simulink model "Speed"  (R2021a)
settings: Solver=ode113  StartTime=0.0  StopTime=1  RelTol=1e-6
model workspace (MAT data in the model file):
  Vdc = 30
  f_pwm = 10000
libraries: pid_lib x7, spsControlledVoltageSourceLib x2, spsGroundLib x2, spsPermanentMagnetSynchronousMachineLib x2, spsThreePhaseVIMeasurementLib x2, spsUniversalBridgeLib x2, spsTriangleGeneratorLib x2, spspowerguiLib x1
settings Model: SimulationMode=accelerator  Creator=Zzx  LastModifiedBy=Zzx
settings SolverCC: ZeroCrossAlgorithm=Adaptive

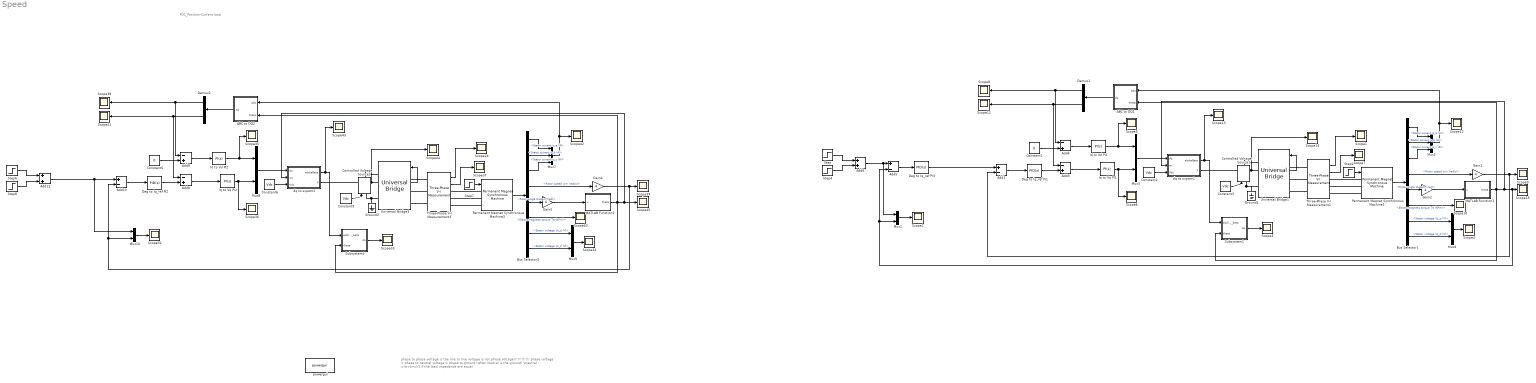
== system Speed ==
  note: FOC_Position-Current loop
  note: phase to phase voltage is the line to line voltage
      | is not phase voltage!!!!!!!!!!!!
      | phase voltage = phase to neutral voltage = phase to ground (when neutral is the ground)
      | Vneutral =(a+b+c)/3 if the load impedance are equal
  ABC to DQ1 : Subsystem
  ABC to DQ2 : Subsystem
  Add1 : Sum  Inputs=+-
  Add10 : Sum  Inputs=+-
  Add11 : Sum
  Add{3..4,8..9} (4 alike) : Sum  Inputs=-+
  Add5 : Sum  Inputs=+-
  Add6 : Sum
  Bus Selector1 : BusSelector  OutputSignals=Stator current is_a (A),Stator current is_b (A),Stator current is_c (A),Rotor speed wm (rad/s),Rotor angle thetam (rad),Electromagnetic torque Te (N*m),Stator voltage Vs_q (V),Stator voltage Vs_d (V)
  Bus Selector3 : BusSelector  OutputSignals=Stator current is_a (A),Stator current is_b (A),Stator current is_c (A),Rotor speed wm (rad/s),Rotor angle thetam (rad),Electromagnetic torque Te (N*m),Stator voltage Vs_q (V),Stator voltage Vs_d (V)
  Constant1 : Constant  Value=0
  Constant{2..3,6,9} (4 alike) : Constant  Value=Vdc
  Constant5 : Constant  Value=0
  Controlled Voltage Source1 : spsControlledVoltageSourceLib/Controlled Voltage Source  Initialize=on  Source_Type=DC  Amplitude=0  Phase=0  Frequency=0  Measurements=Voltage
  Controlled Voltage Source2 : spsControlledVoltageSourceLib/Controlled Voltage Source  Initialize=on  Source_Type=DC  Amplitude=0  Phase=0  Frequency=0  Measurements=Voltage
  Deg to Iq_ref PI1 : pid_lib/PID Controller  Controller=PID  Form=Parallel  TimeDomain=Continuous-time  UseExternalTs=off  SampleTime=-1  IntegratorMethod=Forward Euler  FilterMethod=Forward Euler  ControllerParametersSource=internal  P=80  I=0.1  D=1  UseFilter=on  N=10  TunerSelectOption=Frequency Response Based  InitialConditionSource=internal  InitialConditionForIntegrator=0  InitialConditionForFilter=0  DifferentiatorICPrevScaledInput=0  ExternalReset=none  TrackingMode=off  Kt=1  LimitOutput=off  SatLimitsSource=internal  UpperSaturationLimit=inf  LowerSaturationLimit=-inf  LinearizeAsGain=on  AntiWindupMode=none  Kb=1  POutMin=[]  POutMax=[]  IOutMin=[]  IOutMax=[]  DOutMin=[]  DOutMax=[]  NOutMin=[]  NOutMax=[]  SumOutMin=[]  SumOutMax=[]  SaturationOutMin=[]  SaturationOutMax=[]  PParamMin=[]  PParamMax=[]  IParamMin=[]  IParamMax=[]  DParamMin=[]  DParamMax=[]  NParamMin=[]  NParamMax=[]  KbParamMin=[]  KbParamMax=[]  KtParamMin=[]  KtParamMax=[]  KbOutMin=[]  KbOutMax=[]  KtOutMin=[]  KtOutMax=[]  IntegratorOutMin=[]  IntegratorOutMax=[]  FilterOutMin=[]  FilterOutMax=[]  SumI1OutMin=[]  SumI1OutMax=[]  SumI2OutMin=[]  SumI2OutMax=[]  SumI3OutMin=[]  SumI3OutMax=[]  SumI4OutMin=[]  SumI4OutMax=[]  SumDOutMin=[]  SumDOutMax=[]  DifferentiatorOutMin=[]  DifferentiatorOutMax=[]  FilterDiffOutCoefMin=[]  FilterDiffOutCoefMax=[]  ReciprocalOutMin=[]  ReciprocalOutMax=[]  SumDenOutMin=[]  SumDenOutMax=[]  SumNumOutMin=[]  SumNumOutMax=[]  DivideOutMin=[]  DivideOutMax=[]  UdiffTsProdOutMin=[]  UdiffTsProdOutMax=[]  NTsProdOutMin=[]  NTsProdOutMax=[]  UintegralTsProdOutMin=[]  UintegralTsProdOutMax=[]  UngainTsProdOutMin=[]  UngainTsProdOutMax=[]  IntegratorContinuousStateAttributes=''  IntegratorStateMustResolveToSignalObject=off  IntegratorRTWStateStorageClass=Auto  FilterContinuousStateAttributes=''  FilterStateMustResolveToSignalObject=off  FilterRTWStateStorageClass=Auto  ParallelPVariant=InternalParameters  IdealPVariant=Disabled  IVariant=InternalParameters  DVariant=InternalParameters  IntegratorVariant=Continuous  SatVariant=Disabled  AWVariant=Passthrough  PCopyVariant=Disabled  TRVariant=Disabled  FdbkBlocksVariant=Forward  IdealPFdbkVariant=Disabled  SatFdbkVariant=Disabled  DerivativeFilterVariant=ContFilter  NVariant=InternalParameters  NCopyVariant=Disabled  FilterICVariant=InternalICsFilter  IntegratorICVariant=InternalICs  ExternalResetVariant=Disabled  TRSumVariant=Passthrough  SumFdbkVariant=Disabled  SumVariant=Sum_PID  TsampFilterVariant=InternalTs  TsampNgainVariant=Passthrough  TsampIntegralVariant=Passthrough  ExternalSaturationOutDataTypeStr=Inherit: Same as second input
  Deg to Iq_ref PI2 : pid_lib/PID Controller  Controller=PID  Form=Parallel  TimeDomain=Continuous-time  UseExternalTs=off  SampleTime=-1  IntegratorMethod=Forward Euler  FilterMethod=Forward Euler  ControllerParametersSource=internal  P=80  I=0.1  D=0.1  UseFilter=on  N=10  TunerSelectOption=Frequency Response Based  InitialConditionSource=internal  InitialConditionForIntegrator=0  InitialConditionForFilter=0  DifferentiatorICPrevScaledInput=0  ExternalReset=none  TrackingMode=off  Kt=1  LimitOutput=off  SatLimitsSource=internal  UpperSaturationLimit=inf  LowerSaturationLimit=-inf  LinearizeAsGain=on  AntiWindupMode=none  Kb=1  POutMin=[]  POutMax=[]  IOutMin=[]  IOutMax=[]  DOutMin=[]  DOutMax=[]  NOutMin=[]  NOutMax=[]  SumOutMin=[]  SumOutMax=[]  SaturationOutMin=[]  SaturationOutMax=[]  PParamMin=[]  PParamMax=[]  IParamMin=[]  IParamMax=[]  DParamMin=[]  DParamMax=[]  NParamMin=[]  NParamMax=[]  KbParamMin=[]  KbParamMax=[]  KtParamMin=[]  KtParamMax=[]  KbOutMin=[]  KbOutMax=[]  KtOutMin=[]  KtOutMax=[]  IntegratorOutMin=[]  IntegratorOutMax=[]  FilterOutMin=[]  FilterOutMax=[]  SumI1OutMin=[]  SumI1OutMax=[]  SumI2OutMin=[]  SumI2OutMax=[]  SumI3OutMin=[]  SumI3OutMax=[]  SumI4OutMin=[]  SumI4OutMax=[]  SumDOutMin=[]  SumDOutMax=[]  DifferentiatorOutMin=[]  DifferentiatorOutMax=[]  FilterDiffOutCoefMin=[]  FilterDiffOutCoefMax=[]  ReciprocalOutMin=[]  ReciprocalOutMax=[]  SumDenOutMin=[]  SumDenOutMax=[]  SumNumOutMin=[]  SumNumOutMax=[]  DivideOutMin=[]  DivideOutMax=[]  UdiffTsProdOutMin=[]  UdiffTsProdOutMax=[]  NTsProdOutMin=[]  NTsProdOutMax=[]  UintegralTsProdOutMin=[]  UintegralTsProdOutMax=[]  UngainTsProdOutMin=[]  UngainTsProdOutMax=[]  IntegratorContinuousStateAttributes=''  IntegratorStateMustResolveToSignalObject=off  IntegratorRTWStateStorageClass=Auto  FilterContinuousStateAttributes=''  FilterStateMustResolveToSignalObject=off  FilterRTWStateStorageClass=Auto  ParallelPVariant=InternalParameters  IdealPVariant=Disabled  IVariant=InternalParameters  DVariant=InternalParameters  IntegratorVariant=Continuous  SatVariant=Disabled  AWVariant=Passthrough  PCopyVariant=Disabled  TRVariant=Disabled  FdbkBlocksVariant=Forward  IdealPFdbkVariant=Disabled  SatFdbkVariant=Disabled  DerivativeFilterVariant=ContFilter  NVariant=InternalParameters  NCopyVariant=Disabled  FilterICVariant=InternalICsFilter  IntegratorICVariant=InternalICs  ExternalResetVariant=Disabled  TRSumVariant=Passthrough  SumFdbkVariant=Disabled  SumVariant=Sum_PID  TsampFilterVariant=InternalTs  TsampNgainVariant=Passthrough  TsampIntegralVariant=Passthrough  ExternalSaturationOutDataTypeStr=Inherit: Same as second input
  Deg to Iq_ref PI3 : pid_lib/PID Controller  Controller=PID  Form=Parallel  TimeDomain=Continuous-time  UseExternalTs=off  SampleTime=-1  IntegratorMethod=Forward Euler  FilterMethod=Forward Euler  ControllerParametersSource=internal  P=53  I=2  D=0.8  UseFilter=on  N=10  TunerSelectOption=Frequency Response Based  InitialConditionSource=internal  InitialConditionForIntegrator=0  InitialConditionForFilter=0  DifferentiatorICPrevScaledInput=0  ExternalReset=none  TrackingMode=off  Kt=1  LimitOutput=off  SatLimitsSource=internal  UpperSaturationLimit=inf  LowerSaturationLimit=-inf  LinearizeAsGain=on  AntiWindupMode=none  Kb=1  POutMin=[]  POutMax=[]  IOutMin=[]  IOutMax=[]  DOutMin=[]  DOutMax=[]  NOutMin=[]  NOutMax=[]  SumOutMin=[]  SumOutMax=[]  SaturationOutMin=[]  SaturationOutMax=[]  PParamMin=[]  PParamMax=[]  IParamMin=[]  IParamMax=[]  DParamMin=[]  DParamMax=[]  NParamMin=[]  NParamMax=[]  KbParamMin=[]  KbParamMax=[]  KtParamMin=[]  KtParamMax=[]  KbOutMin=[]  KbOutMax=[]  KtOutMin=[]  KtOutMax=[]  IntegratorOutMin=[]  IntegratorOutMax=[]  FilterOutMin=[]  FilterOutMax=[]  SumI1OutMin=[]  SumI1OutMax=[]  SumI2OutMin=[]  SumI2OutMax=[]  SumI3OutMin=[]  SumI3OutMax=[]  SumI4OutMin=[]  SumI4OutMax=[]  SumDOutMin=[]  SumDOutMax=[]  DifferentiatorOutMin=[]  DifferentiatorOutMax=[]  FilterDiffOutCoefMin=[]  FilterDiffOutCoefMax=[]  ReciprocalOutMin=[]  ReciprocalOutMax=[]  SumDenOutMin=[]  SumDenOutMax=[]  SumNumOutMin=[]  SumNumOutMax=[]  DivideOutMin=[]  DivideOutMax=[]  UdiffTsProdOutMin=[]  UdiffTsProdOutMax=[]  NTsProdOutMin=[]  NTsProdOutMax=[]  UintegralTsProdOutMin=[]  UintegralTsProdOutMax=[]  UngainTsProdOutMin=[]  UngainTsProdOutMax=[]  IntegratorContinuousStateAttributes=''  IntegratorStateMustResolveToSignalObject=off  IntegratorRTWStateStorageClass=Auto  FilterContinuousStateAttributes=''  FilterStateMustResolveToSignalObject=off  FilterRTWStateStorageClass=Auto  ParallelPVariant=InternalParameters  IdealPVariant=Disabled  IVariant=InternalParameters  DVariant=InternalParameters  IntegratorVariant=Continuous  SatVariant=Disabled  AWVariant=Passthrough  PCopyVariant=Disabled  TRVariant=Disabled  FdbkBlocksVariant=Forward  IdealPFdbkVariant=Disabled  SatFdbkVariant=Disabled  DerivativeFilterVariant=ContFilter  NVariant=InternalParameters  NCopyVariant=Disabled  FilterICVariant=InternalICsFilter  IntegratorICVariant=InternalICs  ExternalResetVariant=Disabled  TRSumVariant=Passthrough  SumFdbkVariant=Disabled  SumVariant=Sum_PID  TsampFilterVariant=InternalTs  TsampNgainVariant=Passthrough  TsampIntegralVariant=Passthrough  ExternalSaturationOutDataTypeStr=Inherit: Same as second input
  Demux1 : Demux  Outputs=2
  Demux2 : Demux  Outputs=2
  Gain{1..2,4..5} (4 alike) : Gain  Gain=4
  Ground1 : spsGroundLib/Ground  LConnTagsString=a
  Ground2 : spsGroundLib/Ground  LConnTagsString=a
  Id to Vd PI1 : pid_lib/PID Controller  Controller=PI  Form=Parallel  TimeDomain=Continuous-time  UseExternalTs=off  SampleTime=-1  IntegratorMethod=Forward Euler  FilterMethod=Forward Euler  ControllerParametersSource=internal  P=1  I=0.5  D=0  UseFilter=on  N=100  TunerSelectOption=Transfer Function Based (PID Tuner App)  InitialConditionSource=internal  InitialConditionForIntegrator=0  InitialConditionForFilter=0  DifferentiatorICPrevScaledInput=0  ExternalReset=none  TrackingMode=off  Kt=1  LimitOutput=off  SatLimitsSource=internal  UpperSaturationLimit=inf  LowerSaturationLimit=-inf  LinearizeAsGain=on  AntiWindupMode=none  Kb=1  POutMin=[]  POutMax=[]  IOutMin=[]  IOutMax=[]  DOutMin=[]  DOutMax=[]  NOutMin=[]  NOutMax=[]  SumOutMin=[]  SumOutMax=[]  SaturationOutMin=[]  SaturationOutMax=[]  PParamMin=[]  PParamMax=[]  IParamMin=[]  IParamMax=[]  DParamMin=[]  DParamMax=[]  NParamMin=[]  NParamMax=[]  KbParamMin=[]  KbParamMax=[]  KtParamMin=[]  KtParamMax=[]  KbOutMin=[]  KbOutMax=[]  KtOutMin=[]  KtOutMax=[]  IntegratorOutMin=[]  IntegratorOutMax=[]  FilterOutMin=[]  FilterOutMax=[]  SumI1OutMin=[]  SumI1OutMax=[]  SumI2OutMin=[]  SumI2OutMax=[]  SumI3OutMin=[]  SumI3OutMax=[]  SumI4OutMin=[]  SumI4OutMax=[]  SumDOutMin=[]  SumDOutMax=[]  DifferentiatorOutMin=[]  DifferentiatorOutMax=[]  FilterDiffOutCoefMin=[]  FilterDiffOutCoefMax=[]  ReciprocalOutMin=[]  ReciprocalOutMax=[]  SumDenOutMin=[]  SumDenOutMax=[]  SumNumOutMin=[]  SumNumOutMax=[]  DivideOutMin=[]  DivideOutMax=[]  UdiffTsProdOutMin=[]  UdiffTsProdOutMax=[]  NTsProdOutMin=[]  NTsProdOutMax=[]  UintegralTsProdOutMin=[]  UintegralTsProdOutMax=[]  UngainTsProdOutMin=[]  UngainTsProdOutMax=[]  IntegratorContinuousStateAttributes=''  IntegratorStateMustResolveToSignalObject=off  IntegratorRTWStateStorageClass=Auto  FilterContinuousStateAttributes=''  FilterStateMustResolveToSignalObject=off  FilterRTWStateStorageClass=Auto  ParallelPVariant=InternalParameters  IdealPVariant=Disabled  IVariant=InternalParameters  DVariant=Disabled  IntegratorVariant=Continuous  SatVariant=Disabled  AWVariant=Passthrough  PCopyVariant=Disabled  TRVariant=Disabled  FdbkBlocksVariant=Forward  IdealPFdbkVariant=Disabled  SatFdbkVariant=Disabled  DerivativeFilterVariant=Disabled  NVariant=Disabled  NCopyVariant=Disabled_SignalSpec  FilterICVariant=Disabled  IntegratorICVariant=InternalICs  ExternalResetVariant=Disabled  TRSumVariant=Passthrough  SumFdbkVariant=Disabled  SumVariant=Sum_PI  TsampFilterVariant=InternalTs  TsampNgainVariant=Passthrough  TsampIntegralVariant=Passthrough  ExternalSaturationOutDataTypeStr=Inherit: Same as second input
  Id to Vd PI2 : pid_lib/PID Controller  Controller=PI  Form=Parallel  TimeDomain=Continuous-time  UseExternalTs=off  SampleTime=-1  IntegratorMethod=Forward Euler  FilterMethod=Forward Euler  ControllerParametersSource=internal  P=1  I=0.5  D=0  UseFilter=on  N=100  TunerSelectOption=Transfer Function Based (PID Tuner App)  InitialConditionSource=internal  InitialConditionForIntegrator=0  InitialConditionForFilter=0  DifferentiatorICPrevScaledInput=0  ExternalReset=none  TrackingMode=off  Kt=1  LimitOutput=off  SatLimitsSource=internal  UpperSaturationLimit=inf  LowerSaturationLimit=-inf  LinearizeAsGain=on  AntiWindupMode=none  Kb=1  POutMin=[]  POutMax=[]  IOutMin=[]  IOutMax=[]  DOutMin=[]  DOutMax=[]  NOutMin=[]  NOutMax=[]  SumOutMin=[]  SumOutMax=[]  SaturationOutMin=[]  SaturationOutMax=[]  PParamMin=[]  PParamMax=[]  IParamMin=[]  IParamMax=[]  DParamMin=[]  DParamMax=[]  NParamMin=[]  NParamMax=[]  KbParamMin=[]  KbParamMax=[]  KtParamMin=[]  KtParamMax=[]  KbOutMin=[]  KbOutMax=[]  KtOutMin=[]  KtOutMax=[]  IntegratorOutMin=[]  IntegratorOutMax=[]  FilterOutMin=[]  FilterOutMax=[]  SumI1OutMin=[]  SumI1OutMax=[]  SumI2OutMin=[]  SumI2OutMax=[]  SumI3OutMin=[]  SumI3OutMax=[]  SumI4OutMin=[]  SumI4OutMax=[]  SumDOutMin=[]  SumDOutMax=[]  DifferentiatorOutMin=[]  DifferentiatorOutMax=[]  FilterDiffOutCoefMin=[]  FilterDiffOutCoefMax=[]  ReciprocalOutMin=[]  ReciprocalOutMax=[]  SumDenOutMin=[]  SumDenOutMax=[]  SumNumOutMin=[]  SumNumOutMax=[]  DivideOutMin=[]  DivideOutMax=[]  UdiffTsProdOutMin=[]  UdiffTsProdOutMax=[]  NTsProdOutMin=[]  NTsProdOutMax=[]  UintegralTsProdOutMin=[]  UintegralTsProdOutMax=[]  UngainTsProdOutMin=[]  UngainTsProdOutMax=[]  IntegratorContinuousStateAttributes=''  IntegratorStateMustResolveToSignalObject=off  IntegratorRTWStateStorageClass=Auto  FilterContinuousStateAttributes=''  FilterStateMustResolveToSignalObject=off  FilterRTWStateStorageClass=Auto  ParallelPVariant=InternalParameters  IdealPVariant=Disabled  IVariant=InternalParameters  DVariant=Disabled  IntegratorVariant=Continuous  SatVariant=Disabled  AWVariant=Passthrough  PCopyVariant=Disabled  TRVariant=Disabled  FdbkBlocksVariant=Forward  IdealPFdbkVariant=Disabled  SatFdbkVariant=Disabled  DerivativeFilterVariant=Disabled  NVariant=Disabled  NCopyVariant=Disabled_SignalSpec  FilterICVariant=Disabled  IntegratorICVariant=InternalICs  ExternalResetVariant=Disabled  TRSumVariant=Passthrough  SumFdbkVariant=Disabled  SumVariant=Sum_PI  TsampFilterVariant=InternalTs  TsampNgainVariant=Passthrough  TsampIntegralVariant=Passthrough  ExternalSaturationOutDataTypeStr=Inherit: Same as second input
  Iq to Vq PI1 : pid_lib/PID Controller  Controller=PI  Form=Parallel  TimeDomain=Continuous-time  UseExternalTs=off  SampleTime=-1  IntegratorMethod=Forward Euler  FilterMethod=Forward Euler  ControllerParametersSource=internal  P=1  I=0.5  D=0  UseFilter=on  N=100  TunerSelectOption=Frequency Response Based  InitialConditionSource=internal  InitialConditionForIntegrator=0  InitialConditionForFilter=0  DifferentiatorICPrevScaledInput=0  ExternalReset=none  TrackingMode=off  Kt=1  LimitOutput=off  SatLimitsSource=internal  UpperSaturationLimit=inf  LowerSaturationLimit=-inf  LinearizeAsGain=on  AntiWindupMode=none  Kb=1  POutMin=[]  POutMax=[]  IOutMin=[]  IOutMax=[]  DOutMin=[]  DOutMax=[]  NOutMin=[]  NOutMax=[]  SumOutMin=[]  SumOutMax=[]  SaturationOutMin=[]  SaturationOutMax=[]  PParamMin=[]  PParamMax=[]  IParamMin=[]  IParamMax=[]  DParamMin=[]  DParamMax=[]  NParamMin=[]  NParamMax=[]  KbParamMin=[]  KbParamMax=[]  KtParamMin=[]  KtParamMax=[]  KbOutMin=[]  KbOutMax=[]  KtOutMin=[]  KtOutMax=[]  IntegratorOutMin=[]  IntegratorOutMax=[]  FilterOutMin=[]  FilterOutMax=[]  SumI1OutMin=[]  SumI1OutMax=[]  SumI2OutMin=[]  SumI2OutMax=[]  SumI3OutMin=[]  SumI3OutMax=[]  SumI4OutMin=[]  SumI4OutMax=[]  SumDOutMin=[]  SumDOutMax=[]  DifferentiatorOutMin=[]  DifferentiatorOutMax=[]  FilterDiffOutCoefMin=[]  FilterDiffOutCoefMax=[]  ReciprocalOutMin=[]  ReciprocalOutMax=[]  SumDenOutMin=[]  SumDenOutMax=[]  SumNumOutMin=[]  SumNumOutMax=[]  DivideOutMin=[]  DivideOutMax=[]  UdiffTsProdOutMin=[]  UdiffTsProdOutMax=[]  NTsProdOutMin=[]  NTsProdOutMax=[]  UintegralTsProdOutMin=[]  UintegralTsProdOutMax=[]  UngainTsProdOutMin=[]  UngainTsProdOutMax=[]  IntegratorContinuousStateAttributes=''  IntegratorStateMustResolveToSignalObject=off  IntegratorRTWStateStorageClass=Auto  FilterContinuousStateAttributes=''  FilterStateMustResolveToSignalObject=off  FilterRTWStateStorageClass=Auto  ParallelPVariant=InternalParameters  IdealPVariant=Disabled  IVariant=InternalParameters  DVariant=Disabled  IntegratorVariant=Continuous  SatVariant=Disabled  AWVariant=Passthrough  PCopyVariant=Disabled  TRVariant=Disabled  FdbkBlocksVariant=Forward  IdealPFdbkVariant=Disabled  SatFdbkVariant=Disabled  DerivativeFilterVariant=Disabled  NVariant=Disabled  NCopyVariant=Disabled_SignalSpec  FilterICVariant=Disabled  IntegratorICVariant=InternalICs  ExternalResetVariant=Disabled  TRSumVariant=Passthrough  SumFdbkVariant=Disabled  SumVariant=Sum_PI  TsampFilterVariant=InternalTs  TsampNgainVariant=Passthrough  TsampIntegralVariant=Passthrough  ExternalSaturationOutDataTypeStr=Inherit: Same as second input
  Iq to Vq PI2 : pid_lib/PID Controller  Controller=PI  Form=Parallel  TimeDomain=Continuous-time  UseExternalTs=off  SampleTime=-1  IntegratorMethod=Forward Euler  FilterMethod=Forward Euler  ControllerParametersSource=internal  P=1  I=0.5  D=0  UseFilter=on  N=100  TunerSelectOption=Frequency Response Based  InitialConditionSource=internal  InitialConditionForIntegrator=0  InitialConditionForFilter=0  DifferentiatorICPrevScaledInput=0  ExternalReset=none  TrackingMode=off  Kt=1  LimitOutput=off  SatLimitsSource=internal  UpperSaturationLimit=inf  LowerSaturationLimit=-inf  LinearizeAsGain=on  AntiWindupMode=none  Kb=1  POutMin=[]  POutMax=[]  IOutMin=[]  IOutMax=[]  DOutMin=[]  DOutMax=[]  NOutMin=[]  NOutMax=[]  SumOutMin=[]  SumOutMax=[]  SaturationOutMin=[]  SaturationOutMax=[]  PParamMin=[]  PParamMax=[]  IParamMin=[]  IParamMax=[]  DParamMin=[]  DParamMax=[]  NParamMin=[]  NParamMax=[]  KbParamMin=[]  KbParamMax=[]  KtParamMin=[]  KtParamMax=[]  KbOutMin=[]  KbOutMax=[]  KtOutMin=[]  KtOutMax=[]  IntegratorOutMin=[]  IntegratorOutMax=[]  FilterOutMin=[]  FilterOutMax=[]  SumI1OutMin=[]  SumI1OutMax=[]  SumI2OutMin=[]  SumI2OutMax=[]  SumI3OutMin=[]  SumI3OutMax=[]  SumI4OutMin=[]  SumI4OutMax=[]  SumDOutMin=[]  SumDOutMax=[]  DifferentiatorOutMin=[]  DifferentiatorOutMax=[]  FilterDiffOutCoefMin=[]  FilterDiffOutCoefMax=[]  ReciprocalOutMin=[]  ReciprocalOutMax=[]  SumDenOutMin=[]  SumDenOutMax=[]  SumNumOutMin=[]  SumNumOutMax=[]  DivideOutMin=[]  DivideOutMax=[]  UdiffTsProdOutMin=[]  UdiffTsProdOutMax=[]  NTsProdOutMin=[]  NTsProdOutMax=[]  UintegralTsProdOutMin=[]  UintegralTsProdOutMax=[]  UngainTsProdOutMin=[]  UngainTsProdOutMax=[]  IntegratorContinuousStateAttributes=''  IntegratorStateMustResolveToSignalObject=off  IntegratorRTWStateStorageClass=Auto  FilterContinuousStateAttributes=''  FilterStateMustResolveToSignalObject=off  FilterRTWStateStorageClass=Auto  ParallelPVariant=InternalParameters  IdealPVariant=Disabled  IVariant=InternalParameters  DVariant=Disabled  IntegratorVariant=Continuous  SatVariant=Disabled  AWVariant=Passthrough  PCopyVariant=Disabled  TRVariant=Disabled  FdbkBlocksVariant=Forward  IdealPFdbkVariant=Disabled  SatFdbkVariant=Disabled  DerivativeFilterVariant=Disabled  NVariant=Disabled  NCopyVariant=Disabled_SignalSpec  FilterICVariant=Disabled  IntegratorICVariant=InternalICs  ExternalResetVariant=Disabled  TRSumVariant=Passthrough  SumFdbkVariant=Disabled  SumVariant=Sum_PI  TsampFilterVariant=InternalTs  TsampNgainVariant=Passthrough  TsampIntegralVariant=Passthrough  ExternalSaturationOutDataTypeStr=Inherit: Same as second input
  MATLAB Function1 : MATLAB Function  TreatAsAtomicUnit=on
  MATLAB Function2 : MATLAB Function  TreatAsAtomicUnit=on
  Mux{1,3..4,8..10} (6 alike) : Mux  Inputs=2
  Mux2 : Mux  Inputs=3
  Mux7 : Mux  Inputs=3
  Permanent Magnet Synchronous Machine1 : spsPermanentMagnetSynchronousMachineLib/Permanent Magnet Synchronous Machine  NbPhases=3  FluxDistribution=Sinusoidal  RotorType=Round  MechanicalLoad=Torque Tm  PresetModel=No  ShowDetailedParameters=on  MeasurementBus=off  Resistance=0.89  Inductance=8.5e-3  dqInductances=[8.5e-3,8.5e-3]  La=0.00062  MachineConstant=Voltage Constant (V_peak L-L / krpm)  Flux=0.0056925  VoltageCst=4.13  TorqueCst=0.034155  Flat=120  Mechanical=[ 0.8e-3, 0 4]  PolePairs=4  InitialConditions=[0,0, 0,0]  InitialConditions5ph=[0 0 0 0 0 0]  RefAngle=Aligned with phase A axis (original Park)  IterativeDiscreteModel=Trapezoidal non iterative  TsBlock=-1  TsPowergui=0
  Permanent Magnet Synchronous Machine3 : spsPermanentMagnetSynchronousMachineLib/Permanent Magnet Synchronous Machine  NbPhases=3  FluxDistribution=Sinusoidal  RotorType=Round  MechanicalLoad=Torque Tm  PresetModel=No  ShowDetailedParameters=on  MeasurementBus=off  Resistance=0.89  Inductance=8.5e-3  dqInductances=[8.5e-3,8.5e-3]  La=0.00062  MachineConstant=Voltage Constant (V_peak L-L / krpm)  Flux=0.0056925  VoltageCst=4.13  TorqueCst=0.034155  Flat=120  Mechanical=[ 0.8e-3, 0 4]  PolePairs=4  InitialConditions=[0,0, 0,0]  InitialConditions5ph=[0 0 0 0 0 0]  RefAngle=Aligned with phase A axis (original Park)  IterativeDiscreteModel=Trapezoidal non iterative  TsBlock=-1  TsPowergui=0
  Scope{1..15,24,32..45} (30 alike) : Scope
  Step : Step  Time=0.25  Before=1  After=5  SampleTime=0
  Step2 : Step  Time=0.6  After=0  SampleTime=0
  Step4 : Step  Time=0.75  After=-2  SampleTime=0
  Step6 : Step  Time=0.25  Before=200  After=100  SampleTime=0
  Step7 : Step  Time=0.6  Before=0.2  After=0.05  SampleTime=0
  Step8 : Step  Time=0.75  After=300  SampleTime=0
  Subsystem1 : Subsystem
  Subsystem2 : Subsystem
  Three-Phase V-I Measurement1 : spsThreePhaseVIMeasurementLib/Three-Phase V-I Measurement  VoltageMeasurement=phase-to-ground  SetLabelV=off  LabelV=Vabc  Vpu=off  VpuLL=off  CurrentMeasurement=yes  SetLabelI=off  LabelI=Iabc  Ipu=off  Pbase=100e6  Vbase=500e3  OutputType=Complex  PhasorSimulation=off  PSBequivalent=0
  Three-Phase V-I Measurement3 : spsThreePhaseVIMeasurementLib/Three-Phase V-I Measurement  VoltageMeasurement=phase-to-ground  SetLabelV=off  LabelV=Vabc  Vpu=off  VpuLL=off  CurrentMeasurement=yes  SetLabelI=off  LabelI=Iabc  Ipu=off  Pbase=100e6  Vbase=500e3  OutputType=Complex  PhasorSimulation=off  PSBequivalent=0
  Universal Bridge1 : spsUniversalBridgeLib/Universal Bridge  Arms=3  SnubberResistance=1e5  SnubberCapacitance=inf  Device=IGBT / Diodes  Ron=1e-3  Lon=0  ForwardVoltages="[  0  0  ]"  ForwardVoltage=0  GTOparameters=[ 10e-6 , 20e-6 ]  IGBTparameters=[ 1e-6 , 2e-6 ]  Measurements=None  Measurements_2=None  converterType=Rectifier
  Universal Bridge3 : spsUniversalBridgeLib/Universal Bridge  Arms=3  SnubberResistance=1e5  SnubberCapacitance=inf  Device=IGBT / Diodes  Ron=1e-3  Lon=0  ForwardVoltages="[  0  0  ]"  ForwardVoltage=0  GTOparameters=[ 10e-6 , 20e-6 ]  IGBTparameters=[ 1e-6 , 2e-6 ]  Measurements=None  Measurements_2=None  converterType=Rectifier
  dq to svpwm1 : Subsystem
  dq to svpwm2 : Subsystem
  powergui : spspowerguiLib/powergui  Priority=1  SimulationMode=Continuous  SampleTime=50e-6  frequency=60  Iterations=50  frequencyindice=0  Pbase=100e6  ErrMax=1e-4  UnitsV=kV  UnitsW=MW  buscounter=0  FunctionMessages=off  echomessages=off  EnableUseOfTLC=off  CurrentSourceSwitches=off  DisableSnubberDevices=off  DisableRonSwitches=off  DisableVfSwitches=off  DisplayEquations=off  AutomaticDiscreteSolvers=off  SolverType=Tustin/Backward Euler (TBE)  Interpol=off  ExternalGateDelay=off  methode=off  Ts=100  x0status=blocks  SPID=on  SwTol=0  HookPort=off  NonlinearTolerance=1e-4  nMaxIteration=100  ContinueOnMaxIteration=off  RestoreLinks=warning  ResistiveCurrentMeasurement=off  Frange=[0:2:500]  Ylog=off  Xlog=on  ShowGrid=off  save=off  variable=ZData  structure=0  ZoomFFT=off  StartTime=0.0  cycles=1  DisplayStyle=1  fundamental=60  FreqAxis=off  MaxFrequency=1000  frequencyindicesteady=1  RmsSteady=1  display=off
  wires:
  Constant5/1 -> Add9/2
  Three-Phase V-I Measurement3/1 -> Scope24/1
  Bus Selector3/1 -> Mux7/1  "<Stator current is_a (A)>"
  ABC to DQ2/1(dq) -> Demux2/1
  Mux9/1 -> Scope34/1
  Bus Selector3/3 -> Mux7/3  "<Stator current is_c (A)>"
  Mux7/1 -> ABC to DQ2/1(abc), Scope42/1
  Bus Selector3/8 -> Mux9/2  "<Stator voltage Vs_d (V)>"
  Demux2/2 -> Scope41/1, Add8/1
  Demux2/1 -> Scope38/1, Add9/1
  Bus Selector3/7 -> Mux9/1  "<Stator voltage Vs_q (V)>"
  Bus Selector3/4 -> Gain4/1  "<Rotor speed wm (rad/s)>"
  MATLAB Function2/1(theta) -> Subsystem2/2(theta), ABC to DQ2/2(theta), dq to svpwm2/2(wt), Scope45/1
  Id to Vd PI2/1 -> Scope35/1, Mux8/1
  Bus Selector3/2 -> Mux7/2  "<Stator current is_b (A)>"
  Add9/1 -> Id to Vd PI2/1
  Step7/1 -> Permanent Magnet Synchronous Machine3/1
  Gain4/1 -> Mux10/2, Add10/2, Scope39/1
  Bus Selector3/6 -> Scope40/1  "<Electromagnetic torque Te (N*m)>"
  Add10/1 -> Deg to Iq_ref PI2/1
  Three-Phase V-I Measurement3/2 -> Scope37/1
  Bus Selector3/5 -> Gain5/1  "<Rotor angle thetam (rad)>"
  Permanent Magnet Synchronous Machine3/1 -> Bus Selector3/1
  Mux8/1 -> dq to svpwm2/1(dq)
  Iq to Vq PI2/1 -> Scope36/1, Mux8/2
  Subsystem2/1(dq) -> Scope33/1
  Gain5/1 -> MATLAB Function2/1(u)
  Add8/1 -> Iq to Vq PI2/1
  dq to svpwm2/1(alphaBeta) -> Subsystem2/1(alpha_beta), Scope43/1
  dq to svpwm2/2(P) -> Universal Bridge3/1, Scope44/1
  Constant6/1 -> dq to svpwm2/3(Vdc)
  Step8/1 -> Add11/2
  Step6/1 -> Add11/1
  Constant9/1 -> Controlled Voltage Source2/1
  Deg to Iq_ref PI2/1 -> Add8/2
  Add11/1 -> Mux10/1, Add10/1
  Mux10/1 -> Scope32/1
  Three-Phase V-I Measurement1/1 -> Scope1/1
  Bus Selector1/5 -> Gain2/1  "<Rotor angle thetam (rad)>"
  Demux1/2 -> Scope11/1, Add3/1
  Bus Selector1/6 -> Scope10/1  "<Electromagnetic torque Te (N*m)>"
  Permanent Magnet Synchronous Machine1/1 -> Bus Selector1/1
  Step2/1 -> Permanent Magnet Synchronous Machine1/1
  Subsystem1/1(dq) -> Scope3/1
  Bus Selector1/1 -> Mux2/1  "<Stator current is_a (A)>"
  Demux1/1 -> Scope8/1, Add4/1
  Constant1/1 -> Add4/2
  Mux2/1 -> ABC to DQ1/1(abc), Scope12/1
  Gain1/1 -> Add1/2, Scope9/1
  MATLAB Function1/1(theta) -> Subsystem1/2(theta), ABC to DQ1/2(theta), dq to svpwm1/2(wt), Mux1/2, Add5/2, Scope15/1
  Bus Selector1/3 -> Mux2/3  "<Stator current is_c (A)>"
  Iq to Vq PI1/1 -> Scope6/1, Mux3/2
  Bus Selector1/4 -> Gain1/1  "<Rotor speed wm (rad/s)>"
  Mux3/1 -> dq to svpwm1/1(dq)
  Three-Phase V-I Measurement1/2 -> Scope7/1
  Constant3/1 -> Controlled Voltage Source1/1
  Deg to Iq_ref PI3/1 -> Add1/1
  Add4/1 -> Id to Vd PI1/1
  Bus Selector1/2 -> Mux2/2  "<Stator current is_b (A)>"
  Mux1/1 -> Scope2/1
  Add3/1 -> Iq to Vq PI1/1
  Deg to Iq_ref PI1/1 -> Add3/2
  Mux4/1 -> Scope4/1
  Bus Selector1/8 -> Mux4/2  "<Stator voltage Vs_d (V)>"
  Add1/1 -> Deg to Iq_ref PI1/1
  Constant2/1 -> dq to svpwm1/3(Vdc)
  Gain2/1 -> MATLAB Function1/1(u)
  Bus Selector1/7 -> Mux4/1  "<Stator voltage Vs_q (V)>"
  dq to svpwm1/2(P) -> Universal Bridge1/1, Scope14/1
  dq to svpwm1/1(alphaBeta) -> Subsystem1/1(alpha_beta), Scope13/1
  ABC to DQ1/1(dq) -> Demux1/1
  Id to Vd PI1/1 -> Scope5/1, Mux3/1
  Add5/1 -> Deg to Iq_ref PI3/1
  Add6/1 -> Mux1/1, Add5/1
  Step/1 -> Add6/1
  Step4/1 -> Add6/2
  connections:
  Ground2/LConn1 -- Universal Bridge3/RConn2 -- Controlled Voltage Source2/LConn1
  Permanent Magnet Synchronous Machine3/LConn1 -- Three-Phase V-I Measurement3/RConn1
  Three-Phase V-I Measurement3/LConn1 -- Universal Bridge3/LConn1
  Permanent Magnet Synchronous Machine3/LConn3 -- Three-Phase V-I Measurement3/RConn3
  Three-Phase V-I Measurement3/LConn2 -- Universal Bridge3/LConn2
  Controlled Voltage Source2/RConn1 -- Universal Bridge3/RConn1
  Permanent Magnet Synchronous Machine3/LConn2 -- Three-Phase V-I Measurement3/RConn2
  Three-Phase V-I Measurement3/LConn3 -- Universal Bridge3/LConn3
  Controlled Voltage Source1/LConn1 -- Ground1/LConn1 -- Universal Bridge1/RConn2
  Permanent Magnet Synchronous Machine1/LConn1 -- Three-Phase V-I Measurement1/RConn1
  Three-Phase V-I Measurement1/LConn1 -- Universal Bridge1/LConn1
  Controlled Voltage Source1/RConn1 -- Universal Bridge1/RConn1
  Permanent Magnet Synchronous Machine1/LConn2 -- Three-Phase V-I Measurement1/RConn2
  Three-Phase V-I Measurement1/LConn2 -- Universal Bridge1/LConn2
  Three-Phase V-I Measurement1/LConn3 -- Universal Bridge1/LConn3
  Permanent Magnet Synchronous Machine1/LConn3 -- Three-Phase V-I Measurement1/RConn3

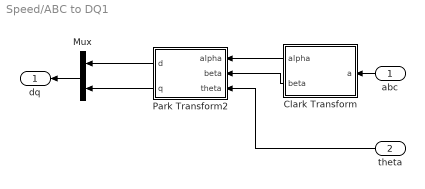
== system Speed/ABC to DQ1 ==
  abc : Inport
  theta : Inport  Port=2
  Clark Transform : MATLAB Function  TreatAsAtomicUnit=on
  Mux : Mux  Inputs=2
  Park Transform2 : MATLAB Function  TreatAsAtomicUnit=on
  dq : Outport
  wires:
  Clark Transform/1(alpha) -> Park Transform2/1(alpha)
  Clark Transform/2(beta) -> Park Transform2/2(beta)
  abc/1 -> Clark Transform/1(a)
  theta/1 -> Park Transform2/3(theta)
  Park Transform2/1(d) -> Mux/1
  Park Transform2/2(q) -> Mux/2
  Mux/1 -> dq/1

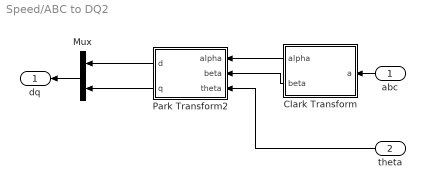
== system Speed/ABC to DQ2 ==
  abc : Inport
  theta : Inport  Port=2
  Clark Transform : MATLAB Function  TreatAsAtomicUnit=on
  Mux : Mux  Inputs=2
  Park Transform2 : MATLAB Function  TreatAsAtomicUnit=on
  dq : Outport
  wires:
  Clark Transform/1(alpha) -> Park Transform2/1(alpha)
  Clark Transform/2(beta) -> Park Transform2/2(beta)
  abc/1 -> Clark Transform/1(a)
  theta/1 -> Park Transform2/3(theta)
  Park Transform2/1(d) -> Mux/1
  Park Transform2/2(q) -> Mux/2
  Mux/1 -> dq/1

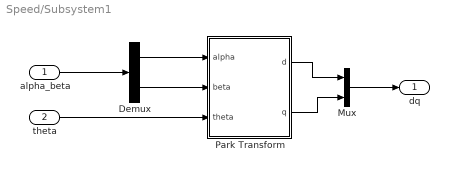
== system Speed/Subsystem1 ==
  alpha_beta : Inport
  theta : Inport  Port=2
  Demux : Demux  Outputs=2
  Mux : Mux  Inputs=2
  Park Transform : MATLAB Function  TreatAsAtomicUnit=on
  dq : Outport
  wires:
  Demux/2 -> Park Transform/2(beta)
  theta/1 -> Park Transform/3(theta)
  Park Transform/1(d) -> Mux/1
  Park Transform/2(q) -> Mux/2
  Mux/1 -> dq/1
  Demux/1 -> Park Transform/1(alpha)
  alpha_beta/1 -> Demux/1

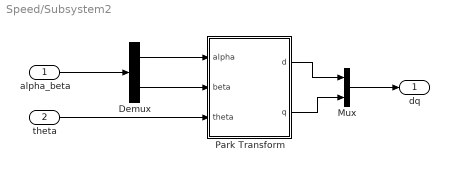
== system Speed/Subsystem2 ==
  alpha_beta : Inport
  theta : Inport  Port=2
  Demux : Demux  Outputs=2
  Mux : Mux  Inputs=2
  Park Transform : MATLAB Function  TreatAsAtomicUnit=on
  dq : Outport
  wires:
  Demux/2 -> Park Transform/2(beta)
  theta/1 -> Park Transform/3(theta)
  Park Transform/1(d) -> Mux/1
  Park Transform/2(q) -> Mux/2
  Mux/1 -> dq/1
  Demux/1 -> Park Transform/1(alpha)
  alpha_beta/1 -> Demux/1

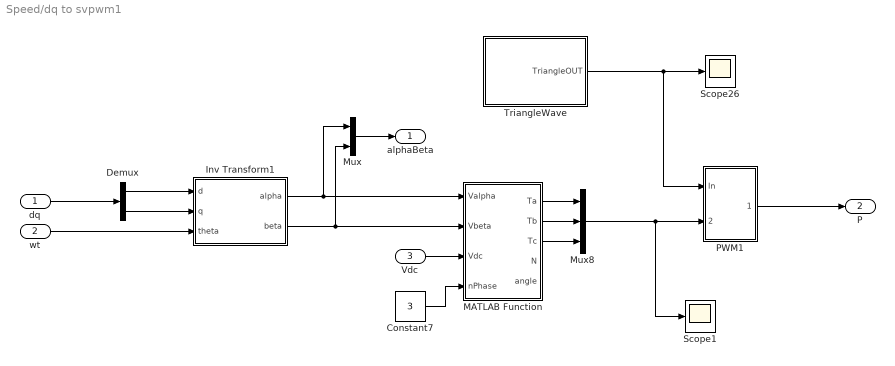
== system Speed/dq to svpwm1 ==
  dq : Inport
  wt : Inport  Port=2
  Vdc : Inport  Port=3
  Constant7 : Constant  Value=3
  Demux : Demux  Outputs=2
  Inv Transform1 : MATLAB Function  TreatAsAtomicUnit=on
  MATLAB Function : MATLAB Function  TreatAsAtomicUnit=on
  Mux : Mux  Inputs=2
  Mux8 : Mux  Inputs=3
  PWM1 : Subsystem
  Scope1 : Scope
  Scope26 : Scope
  TriangleWave : Subsystem
  alphaBeta : Outport
  P : Outport  Port=2
  wires:
  Inv Transform1/2(beta) -> Mux/2, MATLAB Function/2(Vbeta)
  wt/1 -> Inv Transform1/3(theta)
  dq/1 -> Demux/1
  Inv Transform1/1(alpha) -> Mux/1, MATLAB Function/1(Valpha)
  MATLAB Function/1(Ta) -> Mux8/1
  MATLAB Function/3(Tc) -> Mux8/3
  MATLAB Function/2(Tb) -> Mux8/2
  Vdc/1 -> MATLAB Function/3(Vdc)
  Constant7/1 -> MATLAB Function/4(nPhase)
  PWM1/1(PWM) -> P/1
  Mux8/1 -> Scope1/1, PWM1/2(Tcm123)
  Demux/1 -> Inv Transform1/1(d)
  Demux/2 -> Inv Transform1/2(q)
  Mux/1 -> alphaBeta/1
  TriangleWave/1(TriangleOUT) -> Scope26/1, PWM1/1(In)

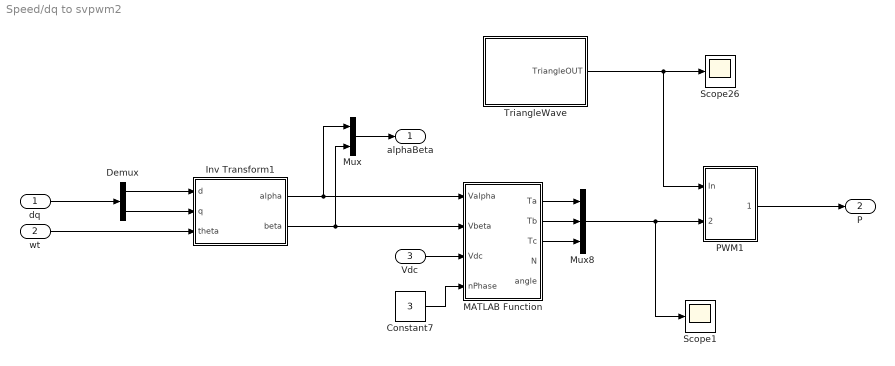
== system Speed/dq to svpwm2 ==
  dq : Inport
  wt : Inport  Port=2
  Vdc : Inport  Port=3
  Constant7 : Constant  Value=3
  Demux : Demux  Outputs=2
  Inv Transform1 : MATLAB Function  TreatAsAtomicUnit=on
  MATLAB Function : MATLAB Function  TreatAsAtomicUnit=on
  Mux : Mux  Inputs=2
  Mux8 : Mux  Inputs=3
  PWM1 : Subsystem
  Scope1 : Scope
  Scope26 : Scope
  TriangleWave : Subsystem
  alphaBeta : Outport
  P : Outport  Port=2
  wires:
  Inv Transform1/2(beta) -> Mux/2, MATLAB Function/2(Vbeta)
  wt/1 -> Inv Transform1/3(theta)
  dq/1 -> Demux/1
  Inv Transform1/1(alpha) -> Mux/1, MATLAB Function/1(Valpha)
  MATLAB Function/1(Ta) -> Mux8/1
  MATLAB Function/3(Tc) -> Mux8/3
  MATLAB Function/2(Tb) -> Mux8/2
  Vdc/1 -> MATLAB Function/3(Vdc)
  Constant7/1 -> MATLAB Function/4(nPhase)
  PWM1/1(PWM) -> P/1
  Mux8/1 -> Scope1/1, PWM1/2(Tcm123)
  Demux/1 -> Inv Transform1/1(d)
  Demux/2 -> Inv Transform1/2(q)
  Mux/1 -> alphaBeta/1
  TriangleWave/1(TriangleOUT) -> Scope26/1, PWM1/1(In)

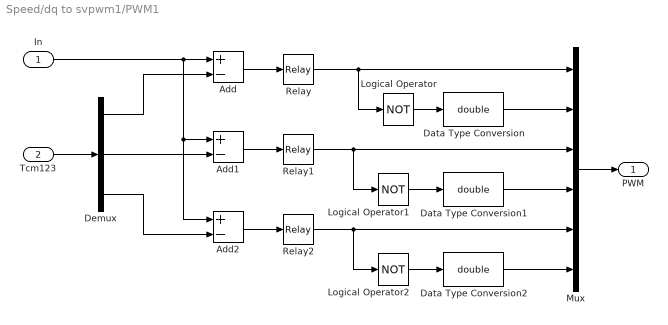
== system Speed/dq to svpwm1/PWM1 ==
  In : Inport
  Tcm123 : Inport  Port=2
  Add : Sum  Inputs=+-
  Add1 : Sum  Inputs=+-
  Add2 : Sum  Inputs=+-
  Data Type Conversion : DataTypeConversion  OutDataTypeStr=double
  Data Type Conversion1 : DataTypeConversion  OutDataTypeStr=double
  Data Type Conversion2 : DataTypeConversion  OutDataTypeStr=double
  Demux : Demux  Outputs=3
  Logical Operator : Logic  Operator=NOT  AllPortsSameDT=off  OutDataTypeStr=boolean
  Logical Operator1 : Logic  Operator=NOT  AllPortsSameDT=off  OutDataTypeStr=boolean
  Logical Operator2 : Logic  Operator=NOT  AllPortsSameDT=off  OutDataTypeStr=boolean
  Mux : Mux  Inputs=6
  Relay : Relay
  Relay1 : Relay
  Relay2 : Relay
  PWM : Outport
  wires:
  Demux/3 -> Add2/2
  Demux/2 -> Add1/2
  Demux/1 -> Add/2
  Relay2/1 -> Mux/5, Logical Operator2/1
  Relay1/1 -> Mux/3, Logical Operator1/1
  Relay/1 -> Logical Operator/1, Mux/1
  Mux/1 -> PWM/1
  Data Type Conversion/1 -> Mux/2
  Data Type Conversion1/1 -> Mux/4
  Data Type Conversion2/1 -> Mux/6
  Logical Operator2/1 -> Data Type Conversion2/1
  Logical Operator1/1 -> Data Type Conversion1/1
  Logical Operator/1 -> Data Type Conversion/1
  Add1/1 -> Relay1/1
  Add2/1 -> Relay2/1
  Add/1 -> Relay/1
  In/1 -> Add/1, Add2/1, Add1/1
  Tcm123/1 -> Demux/1

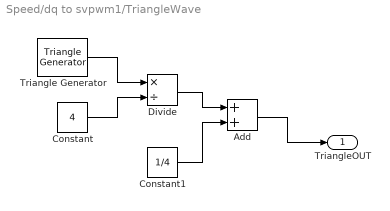
== system Speed/dq to svpwm1/TriangleWave ==
  Add : Sum
  Constant : Constant  Value=4
  Constant1 : Constant  Value=1/4
  Divide : Product  Inputs=*/
  Triangle Generator : spsTriangleGeneratorLib/Triangle Generator  Freq=f_pwm  Phase=90  Ts=0
  TriangleOUT : Outport
  wires:
  Add/1 -> TriangleOUT/1
  Constant/1 -> Divide/2
  Constant1/1 -> Add/2
  Divide/1 -> Add/1
  Triangle Generator/1 -> Divide/1

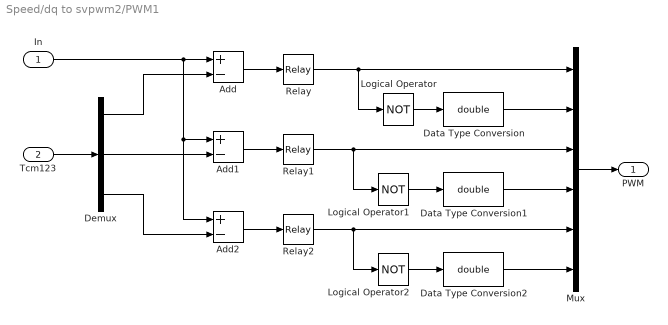
== system Speed/dq to svpwm2/PWM1 ==
  In : Inport
  Tcm123 : Inport  Port=2
  Add : Sum  Inputs=+-
  Add1 : Sum  Inputs=+-
  Add2 : Sum  Inputs=+-
  Data Type Conversion : DataTypeConversion  OutDataTypeStr=double
  Data Type Conversion1 : DataTypeConversion  OutDataTypeStr=double
  Data Type Conversion2 : DataTypeConversion  OutDataTypeStr=double
  Demux : Demux  Outputs=3
  Logical Operator : Logic  Operator=NOT  AllPortsSameDT=off  OutDataTypeStr=boolean
  Logical Operator1 : Logic  Operator=NOT  AllPortsSameDT=off  OutDataTypeStr=boolean
  Logical Operator2 : Logic  Operator=NOT  AllPortsSameDT=off  OutDataTypeStr=boolean
  Mux : Mux  Inputs=6
  Relay : Relay
  Relay1 : Relay
  Relay2 : Relay
  PWM : Outport
  wires:
  Demux/3 -> Add2/2
  Demux/2 -> Add1/2
  Demux/1 -> Add/2
  Relay2/1 -> Mux/5, Logical Operator2/1
  Relay1/1 -> Mux/3, Logical Operator1/1
  Relay/1 -> Logical Operator/1, Mux/1
  Mux/1 -> PWM/1
  Data Type Conversion/1 -> Mux/2
  Data Type Conversion1/1 -> Mux/4
  Data Type Conversion2/1 -> Mux/6
  Logical Operator2/1 -> Data Type Conversion2/1
  Logical Operator1/1 -> Data Type Conversion1/1
  Logical Operator/1 -> Data Type Conversion/1
  Add1/1 -> Relay1/1
  Add2/1 -> Relay2/1
  Add/1 -> Relay/1
  In/1 -> Add/1, Add2/1, Add1/1
  Tcm123/1 -> Demux/1

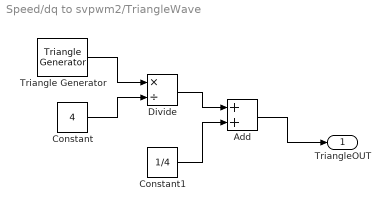
== system Speed/dq to svpwm2/TriangleWave ==
  Add : Sum
  Constant : Constant  Value=4
  Constant1 : Constant  Value=1/4
  Divide : Product  Inputs=*/
  Triangle Generator : spsTriangleGeneratorLib/Triangle Generator  Freq=f_pwm  Phase=90  Ts=0
  TriangleOUT : Outport
  wires:
  Add/1 -> TriangleOUT/1
  Constant/1 -> Divide/2
  Constant1/1 -> Add/2
  Divide/1 -> Add/1
  Triangle Generator/1 -> Divide/1

== matlab function Speed/dq to svpwm2/Inv Transform1 ==
  data: d input; q input; alpha output; theta input; beta output
function [alpha,beta] = fcn(d,q,theta)

alpha = d*cos(theta)-q*sin(theta);
beta = d*sin(theta)+q*cos(theta);

== matlab function Speed/dq to svpwm2/MATLAB Function ==
  data: Valpha input; Ta output; Vbeta input; Vdc input; nPhase input; Tb output; Tc output; N output; angle output
function [Ta, Tb, Tc, N,angle ] = FindT(Valpha, Vbeta, Vdc, nPhase)
% from Valpha Vbeta calculates the 
% T0 - the idle time
% T1 - the time at Vi
% T2 - the time at V(i+1) = Vj

nPhase = floor(nPhase);
if nPhase <3
    nPhase = 3;
end

Valpha = Valpha / Vdc;
Vbeta = Vbeta/Vdc;

angle = atan(Vbeta/Valpha);
if Valpha<0
    angle = angle + pi;
end
if angle <0
    angle = angle + 2*pi;
end

i = floor(angle/pi*nPhase);
Vi = exp(1j*pi*i/nPhase);
Vj = exp(1j*pi*(i+1)/nPhase);

Vm = (Vi+Vj)/2;
Vmabs = abs(Vm);
Vout = Valpha + 1j*Vbeta;
%Vabs = abs(Vout);

Vout_para = real(Vout * conj(Vm))/Vmabs;
if Vout_para > Vmabs
    Vout = Vout /Vout_para *Vmabs;
    Vout_para  = Vmabs;
end

T0 = 1- Vout_para / Vmabs;
Vom = Vout / Vout_para *Vmabs - Vm;
T2 = (real(Vom/(Vj-Vi))+0.5) * (1-T0);
T1 = 1-T0-T2;
N = mod(i,2*nPhase);


Tall = [T0/4 T1/2+T0/4 T2/2+T0/4 T1/2+T2/2+T0/4];

switch (N)
case 0
    Ta = Tall(1);
    Tb = Tall(2);
    Tc = Tall(4);
case 1
    Ta = Tall(3);
    Tb = Tall(1);
    Tc = Tall(4);
case 2
    Ta = Tall(4);
    Tb = Tall(1);
    Tc = Tall(2);
case 3
    Ta = Tall(4);
    Tb = Tall(3);
    Tc = Tall(1);
case 4
    Ta = Tall(2);
    Tb = Tall(4);
    Tc = Tall(1);
case 5
    Ta = Tall(1);
    Tb = Tall(4);
    Tc = Tall(3);
otherwise
    Ta = 0;
    Tb = 0;
    Tc = 0;
            
end

end

== matlab function Speed/ABC to DQ1/Clark Transform ==
  data: a input; alpha output; beta output
function [alpha,beta] = fcn(a)

alpha = a(1)-0.5*a(2)-0.5*a(3);
beta = 0.5*sqrt(3)*a(2)-0.5*sqrt(3)*a(3);

== matlab function Speed/ABC to DQ1/Park Transform2 ==
  data: alpha input; d output; beta input; theta input; q output
function [d,q] = fcn(alpha,beta,theta)

d = alpha*cos(theta)+beta*sin(theta);
q = -alpha*sin(theta)+beta*cos(theta);

== matlab function Speed/MATLAB Function1 ==
  data: u input; theta output
function theta = fcn(u)

theta = mod(u,2*pi);

== matlab function Speed/Subsystem1/Park Transform ==
  data: alpha input; d output; beta input; theta input; q output
function [d,q] = fcn(alpha,beta,theta)

d = alpha*cos(theta)+beta*sin(theta);
q = -alpha*sin(theta)+beta*cos(theta);

== matlab function Speed/dq to svpwm1/Inv Transform1 ==
  data: d input; q input; alpha output; theta input; beta output
function [alpha,beta] = fcn(d,q,theta)

alpha = d*cos(theta)-q*sin(theta);
beta = d*sin(theta)+q*cos(theta);

== matlab function Speed/dq to svpwm1/MATLAB Function ==
  data: Valpha input; Ta output; Vbeta input; Vdc input; nPhase input; Tb output; Tc output; N output; angle output
function [Ta, Tb, Tc, N,angle ] = FindT(Valpha, Vbeta, Vdc, nPhase)
% from Valpha Vbeta calculates the 
% T0 - the idle time
% T1 - the time at Vi
% T2 - the time at V(i+1) = Vj

nPhase = floor(nPhase);
if nPhase <3
    nPhase = 3;
end

Valpha = Valpha / Vdc;
Vbeta = Vbeta/Vdc;

angle = atan(Vbeta/Valpha);
if Valpha<0
    angle = angle + pi;
end
if angle <0
    angle = angle + 2*pi;
end

i = floor(angle/pi*nPhase);
Vi = exp(1j*pi*i/nPhase);
Vj = exp(1j*pi*(i+1)/nPhase);

Vm = (Vi+Vj)/2;
Vmabs = abs(Vm);
Vout = Valpha + 1j*Vbeta;
%Vabs = abs(Vout);

Vout_para = real(Vout * conj(Vm))/Vmabs;
if Vout_para > Vmabs
    Vout = Vout /Vout_para *Vmabs;
    Vout_para  = Vmabs;
end

T0 = 1- Vout_para / Vmabs;
Vom = Vout / Vout_para *Vmabs - Vm;
T2 = (real(Vom/(Vj-Vi))+0.5) * (1-T0);
T1 = 1-T0-T2;
N = mod(i,2*nPhase);


Tall = [T0/4 T1/2+T0/4 T2/2+T0/4 T1/2+T2/2+T0/4];

switch (N)
case 0
    Ta = Tall(1);
    Tb = Tall(2);
    Tc = Tall(4);
case 1
    Ta = Tall(3);
    Tb = Tall(1);
    Tc = Tall(4);
case 2
    Ta = Tall(4);
    Tb = Tall(1);
    Tc = Tall(2);
case 3
    Ta = Tall(4);
    Tb = Tall(3);
    Tc = Tall(1);
case 4
    Ta = Tall(2);
    Tb = Tall(4);
    Tc = Tall(1);
case 5
    Ta = Tall(1);
    Tb = Tall(4);
    Tc = Tall(3);
otherwise
    Ta = 0;
    Tb = 0;
    Tc = 0;
            
end

end

== matlab function Speed/ABC to DQ2/Clark Transform ==
  data: a input; alpha output; beta output
function [alpha,beta] = fcn(a)

alpha = a(1)-0.5*a(2)-0.5*a(3);
beta = 0.5*sqrt(3)*a(2)-0.5*sqrt(3)*a(3);

== matlab function Speed/ABC to DQ2/Park Transform2 ==
  data: alpha input; d output; beta input; theta input; q output
function [d,q] = fcn(alpha,beta,theta)

d = alpha*cos(theta)+beta*sin(theta);
q = -alpha*sin(theta)+beta*cos(theta);

== matlab function Speed/MATLAB Function2 ==
  data: u input; theta output
function theta = fcn(u)

theta = mod(u,2*pi);

== matlab function Speed/Subsystem2/Park Transform ==
  data: alpha input; d output; beta input; theta input; q output
function [d,q] = fcn(alpha,beta,theta)

d = alpha*cos(theta)+beta*sin(theta);
q = -alpha*sin(theta)+beta*cos(theta);
